simulink model "week1_problem2"  (R2020b)
settings: Solver=VariableStepAuto  StartTime=0.0  StopTime=100.0  RelTol=1e-3
model workspace (MAT data in the model file):
  B = Simulink.Parameter
  B.Value = 400
  B.DataType = 'auto'
  B.Dimensions = [1 1]
  K1 = Simulink.Parameter
  K1.Value = 1000
  K1.DataType = 'auto'
  K1.Dimensions = [1 1]
  K2 = Simulink.Parameter
  K2.Value = 960
  K2.DataType = 'auto'
  K2.Dimensions = [1 1]
  M1 = Simulink.Parameter
  M1.Value = 7000
  M1.DataType = 'auto'
  M1.Dimensions = [1 1]
  M2 = Simulink.Parameter
  M2.Value = 250
  M2.DataType = 'auto'
  M2.Dimensions = [1 1]
  h2r = Simulink.Parameter
  h2r.Value = 6.28318530718
  h2r.DataType = 'auto'
  h2r.Dimensions = [1 1]
settings Model: OrderedModelArguments=off  Creator=gokul  LastModifiedBy=gokul
settings DebuggingCC: AlgebraicLoopMsg=none

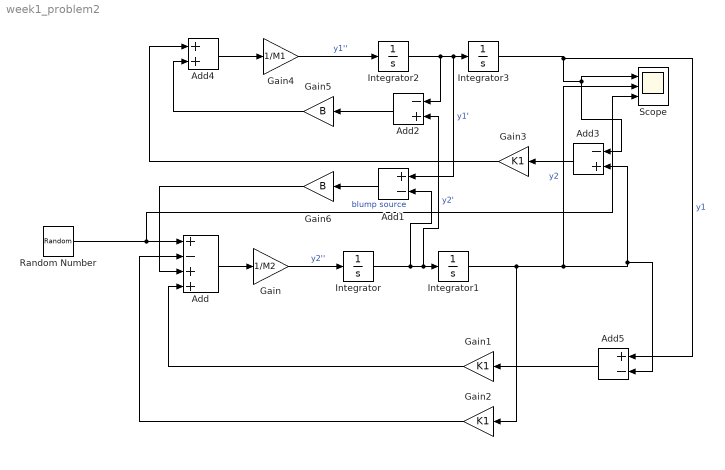
== system week1_problem2 ==
  Add : Sum  Inputs=+-++
  Add1 : Sum  Inputs=+-
  Add2 : Sum  Inputs=-+
  Add3 : Sum  Inputs=-+
  Add4 : Sum
  Add5 : Sum  Inputs=+-
  Gain : Gain  Gain=1/M2
  Gain1 : Gain  Gain=K1
  Gain2 : Gain  Gain=K1
  Gain3 : Gain  Gain=K1
  Gain4 : Gain  Gain=1/M1
  Gain5 : Gain  Gain=B
  Gain6 : Gain  Gain=B
  Integrator{,1..3} (4 alike) : Integrator
  Random Number : RandomNumber  SampleTime=0.1
  Scope : Scope  NumInputPorts=3
  wires:
  Random Number/1 -> Scope/3, Add/1  "blump source"
  Add/1 -> Gain/1
  Gain/1 -> Integrator/1  "y2''"
  Integrator/1 -> Add1/2, Add2/2, Integrator1/1  "y2'"
  Add4/1 -> Gain4/1
  Gain4/1 -> Integrator2/1  "y1''"
  Integrator2/1 -> Add2/1, Add1/1, Integrator3/1  "y1'"
  Integrator3/1 -> Add5/1, Add3/1, Scope/1  "y1"
  Add2/1 -> Gain5/1
  Add1/1 -> Gain6/1
  Gain6/1 -> Add/3
  Gain2/1 -> Add/2
  Gain1/1 -> Add/4
  Integrator1/1 -> Add5/2, Add3/2, Scope/2, Gain2/1  "y2"
  Add5/1 -> Gain1/1
  Add3/1 -> Gain3/1
  Gain3/1 -> Add4/1
  Gain5/1 -> Add4/2
